simulink model "Rate_adaptivity"  (R2022a)
settings: Solver=FixedStepAuto  StartTime=0.0  StopTime=10.0  FixedStep=1e-3  RelTol=1e-3  EnableMultiTasking=on
undefined symbols (not defined in the file): D0, D1, magnitude, PTC16, PTC17
libraries: etargetslib x30, frdmk64flib x5, dspstat3 x1, simulink x1
settings Model: ExtModeTrigDuration=5  Creator=12791  LastModifiedBy=simll
settings OptimizationCC: EnhancedBackFolding=on  PassReuseOutputArgsAs=Individual arguments  ZeroExternalMemoryAtStartup=off  ZeroInternalMemoryAtStartup=off  MaxStackSize=64  OptimizeBlockOrder=speed  DifferentSizesBufferReuse=on  OptimizationCustomize=off  EfficientTunableParamExpr=on
settings DebuggingCC: ParameterTunabilityLossMsg=error
settings HardwareCC: ProdBitPerPointer=32  ProdBitPerSizeT=32  ProdBitPerPtrDiffT=32  ProdLargestAtomicInteger=Long  ProdLargestAtomicFloat=Double  ProdWordSize=32  ProdHWDeviceType=ARM Compatible->ARM Cortex
settings SFSimCC: MATLABDynamicMemAlloc=off
settings RTWCC: SystemTargetFile=ert.tlc  HardwareBoard=NXP FRDM-K64F  TLCOptions="-aInlineSetEventsForThisBaseRateFcn=TLC_FALSE -aSuppressMultiTaskScheduler=TLC_FALSE  -aRateBasedStepFcn=0"  TemplateMakefile=ert_default_tmf  Toolchain=GNU Tools for ARM Embedded Processors
settings CodeAppCC: ForceParamTrailComments=on  IgnoreCustomStorageClasses=off  OperatorAnnotations=on  SimulinkDataObjDesc=on  SFDataObjDesc=on  InsertBlockDesc=on
settings ERTTargetCC: ExtModeTransport=4  ExtModeMexFile=sendToCommService

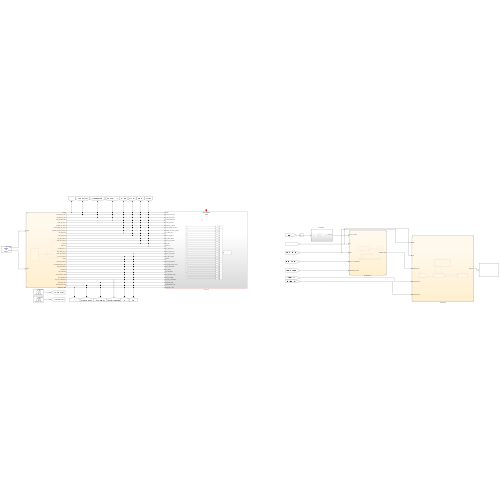
[thumbnail: Simulink's stored preview of the top-level diagram]
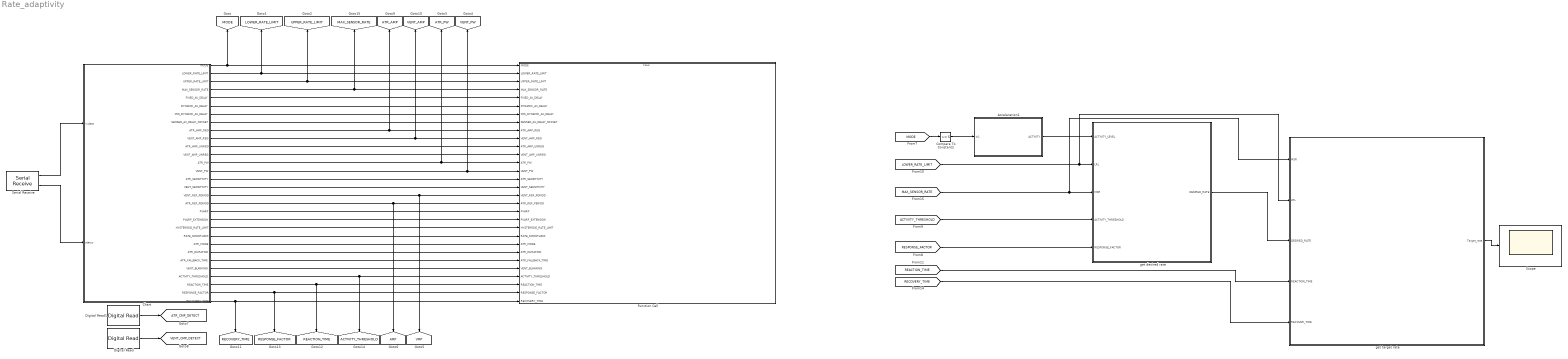
== system Rate_adaptivity ==
  Acceleration1 : Subsystem
  Chart : Stateflow chart  TreatAsAtomicUnit=on
  Compare To Constant2 : simulink/Logic and Bit Operations/Compare To Constant  relop=>=  const=5  OutDataTypeStr=boolean
  Digital Read : frdmk64flib/Digital Read  Whichpin=PTC17 (D1)  SampleTime=-1
  Digital Read1 : frdmk64flib/Digital Read  Whichpin=PTC16 (D0)  SampleTime=-1
  Function Call : Subsystem  TreatAsAtomicUnit=on
  Scope : Scope
  Serial Receive : frdmk64flib/Serial Receive  SCIModule=0  Baudrate=uint32(9600)  Parity=None  StopBits=1  HardwareFlowControl=None  ByteOrder=LittleEndian  DataType=uint8  DataLength=10  BlockingMode=off  OutputStatus=on  SampleTime=0.1
  get desired rate : Stateflow chart  TreatAsAtomicUnit=on
  get target rate : Stateflow chart  TreatAsAtomicUnit=on
      settings: PortSchema="{\"entries\":[{\"content\":{\"sides\":[{\"content\":{\"connectorIds\":[\"In3\",\"In2\",\"In1\",\"In4\",\"In5\"]},\"type\":\"ConnectorPlacement.EquallySpacedRectSide\",\"uuid\":\"b1115713-3752-47d5-be72-104b51cdb1c5\"},{\"content\":{\"connectorIds\":[\"Out1\"],\"side\":\"RIGHT\"},\"type\":\"ConnectorPlacement.EquallySpacedRectSide\",\"uuid\":\"0930a30a-8aa5-4912-ba1f-cc7f148656b0\"},{\"content\":{\"connectorIds\":[],\"side\":\"TOP\"},\"type\":\"ConnectorPlacement.EquallySpacedRectSide\",\"uuid\":\"94dfeeb6-c083-4dc2-b4f5-32fe99d16bb7\"}]},\"type\":\"ConnectorPlacement.EquallySpacedConnector\",\"uuid\":\"5d93a560-4d98-406a-ad12-5273aac4a25c\"}],\"packageUris\":[\"http://schema.mathworks.com/mf0/Connector/R2020b\"],\"version\":\"1.0\"}"
  tag scope: ACTIVITY_THRESHOLD=global, ARP=global, ATR_AMP=global, ATR_CMP_DETECT=global, ATR_PW=global, LOWER_RATE_LIMIT=global, MAX_SENSOR_RATE=global, MODE=global, REACTION_TIME=global, RECOVERY_TIME=global, RESPONSE_FACTOR=global, UPPER_RATE_LIMIT=global, VENT_AMP=global, VENT_CMP_DETECT=global, VENT_PW=global, VRP=global
  wires:
  Serial Receive/1 -> Chart/1(rxdata)
  Serial Receive/2 -> Chart/2(status)
  Chart/1(MODE) -> Function Call/1(MODE), [MODE]
  Chart/2(LOWER_RATE_LIMIT) -> Function Call/2(LOWER_RATE_LIMIT), [LOWER_RATE_LIMIT]
  Chart/3(UPPER_RATE_LIMIT) -> Function Call/3(UPPER_RATE_LIMIT), [UPPER_RATE_LIMIT]
  Chart/4(MAX_SENSOR_RATE) -> Function Call/4(MAX_SENSOR_RATE), [MAX_SENSOR_RATE]
  Chart/5(FIXED_AV_DELAY) -> Function Call/5(FIXED_AV_DELAY)
  Chart/6(DYNAMIC_AV_DELAY) -> Function Call/6(DYNAMIC_AV_DELAY)
  Chart/7(MIN_DYNAMIC_AV_DELAY) -> Function Call/7(MIN_DYNAMIC_AV_DELAY)
  Chart/8(SENSED_AV_DELAY_OFFSET) -> Function Call/8(SENSED_AV_DELAY_OFFSET)
  Chart/11(ATR_AMP_UNREG) -> Function Call/11(ATR_AMP_UNREG)
  Chart/12(VENT_AMP_UNREG) -> Function Call/12(VENT_AMP_UNREG)
  Chart/13(ATR_PW) -> Function Call/13(ATR_PW), [ATR_PW]
  Chart/14(VENT_PW) -> Function Call/14(VENT_PW), [VENT_PW]
  Chart/15(ATR_SENSITIVITY) -> Function Call/15(ATR_SENSITIVITY)
  Chart/16(VENT_SENSITIVITY) -> Function Call/16(VENT_SENSITIVITY)
  Chart/17(VENT_REF_PERIOD) -> Function Call/17(VENT_REF_PERIOD), [VRP]
  Chart/18(ATR_REF_PERIOD) -> Function Call/18(ATR_REF_PERIOD), [ARP]
  Chart/19(PVARP) -> Function Call/19(PVARP)
  Chart/20(PVARP_EXTENSION) -> Function Call/20(PVARP_EXTENSION)
  Chart/21(HYSTERESIS_RATE_LIMIT) -> Function Call/21(HYSTERESIS_RATE_LIMIT)
  Chart/22(RATE_SMOOTHING) -> Function Call/22(RATE_SMOOTHING)
  Chart/23(ATR_MODE) -> Function Call/23(ATR_MODE)
  Chart/24(ATR_DURATION) -> Function Call/24(ATR_DURATION)
  Chart/25(ATR_FALLBACK_TIME) -> Function Call/25(ATR_FALLBACK_TIME)
  Chart/26(VENT_BLANKING) -> Function Call/26(VENT_BLANKING)
  Chart/27(ACTIVITY_THRESHOLD) -> [ACTIVITY_THRESHOLD], Function Call/27(ACTIVITY_THRESHOLD)
  Chart/29(RESPONSE_FACTOR) -> Function Call/29(RESPONSE_FACTOR), [RESPONSE_FACTOR]
  Chart/30(RECOVERY_TIME) -> Function Call/30(RECOVERY_TIME), [RECOVERY_TIME]
  Digital Read1/1 -> [ATR_CMP_DETECT]
  Digital Read/1 -> [VENT_CMP_DETECT]
  Chart/10(VENT_AMP_REG) -> Function Call/10(VENT_AMP_REG), [VENT_AMP]
  Chart/9(ATR_AMP_REG) -> Function Call/9(ATR_AMP_REG), [ATR_AMP]
  Chart/28(REACTION_TIME) -> Function Call/28(REACTION_TIME), [REACTION_TIME]
  [MODE] -> Compare To Constant2/1
  Compare To Constant2/1 -> Acceleration1/1(In1)
  Acceleration1/1(ACTIVITY) -> get desired rate/1(ACTIVITY_LEVEL)
  [LOWER_RATE_LIMIT] -> get desired rate/2(LRL), get target rate/2(LRL)
  [MAX_SENSOR_RATE] -> get desired rate/3(MSR), get target rate/3(MSR)
  [ACTIVITY_THRESHOLD] -> get desired rate/4(ACTIVITY_THRESHOLD)
  [RESPONSE_FACTOR] -> get desired rate/5(RESPONSE_FACTOR)
  get desired rate/1(DESIRED_RATE) -> get target rate/1(DESIRED_RATE)
  [REACTION_TIME] -> get target rate/4(REACTION_TIME)
  [RECOVERY_TIME] -> get target rate/5(RECOVER_TIME)
  get target rate/1(Target_rate) -> Scope/1

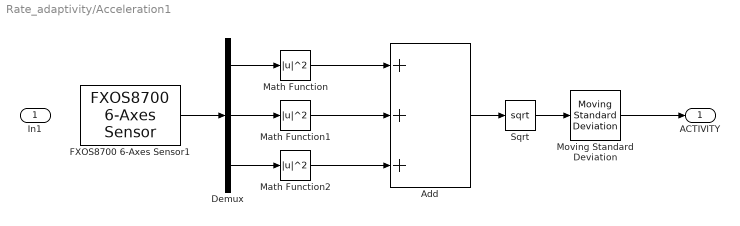
== system Rate_adaptivity/Acceleration1 ==
  In1 : Inport
  Add : Sum  Inputs=+++
  Demux : Demux  Outputs=3
  FXOS8700 6-Axes Sensor1 : frdmk64flib/FXOS8700 6-Axes Sensor  Activesensor=Accelerometer only  ODR=800Hz  HybridODR=400Hz  Accelfullrange=-4g to +4g  SampleTime=-1
  Math Function : Math  Operator=magnitude^2  SignedPower=on  OutDataTypeStr=double
  Math Function1 : Math  Operator=magnitude^2  SignedPower=on  OutDataTypeStr=double
  Math Function2 : Math  Operator=magnitude^2  SignedPower=on  OutDataTypeStr=double
  Moving Standard Deviation : dspstat3/Moving Standard Deviation  Method=Sliding window  ForgettingFactorPort=off  SpecifyWindowLength=on  WindowLength=4  ForgettingFactor=0.9  SimulateUsing=Code generation
      settings: SourceProductBaseCode=DS
  Sqrt : Sqrt
  ACTIVITY : Outport  SourceOfInitialOutputValue=Input signal
  wires:
  Sqrt/1 -> Moving Standard Deviation/1
  Math Function2/1 -> Add/3
  Add/1 -> Sqrt/1
  Math Function1/1 -> Add/2
  Demux/1 -> Math Function/1
  Demux/2 -> Math Function1/1
  Math Function/1 -> Add/1
  FXOS8700 6-Axes Sensor1/1 -> Demux/1
  Demux/3 -> Math Function2/1
  Moving Standard Deviation/1 -> ACTIVITY/1

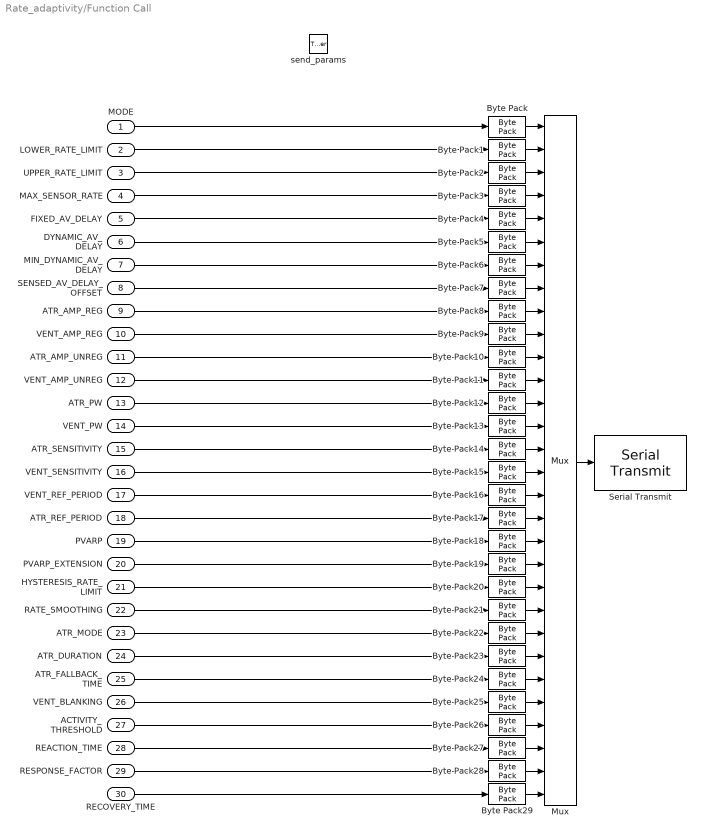
== system Rate_adaptivity/Function Call ==
  MODE : Inport
  LOWER_RATE_LIMIT : Inport  Port=2
  UPPER_RATE_LIMIT : Inport  Port=3
  MAX_SENSOR_RATE : Inport  Port=4
  FIXED_AV_DELAY : Inport  Port=5
  DYNAMIC_AV_DELAY : Inport  Port=6
  MIN_DYNAMIC_AV_DELAY : Inport  Port=7
  SENSED_AV_DELAY_OFFSET : Inport  Port=8
  ATR_AMP_REG : Inport  Port=9
  VENT_AMP_REG : Inport  Port=10
  ATR_AMP_UNREG : Inport  Port=11
  VENT_AMP_UNREG : Inport  Port=12
  ATR_PW : Inport  Port=13
  VENT_PW : Inport  Port=14
  ATR_SENSITIVITY : Inport  Port=15
  VENT_SENSITIVITY : Inport  Port=16
  VENT_REF_PERIOD : Inport  Port=17
  ATR_REF_PERIOD : Inport  Port=18
  PVARP : Inport  Port=19
  PVARP_EXTENSION : Inport  Port=20
  HYSTERESIS_RATE_LIMIT : Inport  Port=21
  RATE_SMOOTHING : Inport  Port=22
  ATR_MODE : Inport  Port=23
  ATR_DURATION : Inport  Port=24
  ATR_FALLBACK_TIME : Inport  Port=25
  VENT_BLANKING : Inport  Port=26
  ACTIVITY_THRESHOLD : Inport  Port=27
  REACTION_TIME : Inport  Port=28
  RESPONSE_FACTOR : Inport  Port=29
  RECOVERY_TIME : Inport  Port=30
  send_params : TriggerPort  TriggerType=function-call  IsSimulinkFunction=on  FunctionName=send_params  VariantControl=Variant
  Byte Pack{,1..4,6..7,16..21,23..25,27..29} (19 alike) : etargetslib/Byte Pack  datatypes={'uint16'}  byteAlign=1
  Byte Pack{8..15,26} (9 alike) : etargetslib/Byte Pack  datatypes={'double'}  byteAlign=1
  Byte Pack22 : etargetslib/Byte Pack  datatypes={'boolean'}  byteAlign=1
  Byte Pack5 : etargetslib/Byte Pack  datatypes={'boolean'}  byteAlign=1
  Mux : Mux  Inputs=30
  Serial Transmit : frdmk64flib/Serial Transmit  SCIModule=0  Baudrate=uint32(9600)  Parity=None  StopBits=1  HardwareFlowControl=None  ByteOrder=LittleEndian  BlockingMode=on  OutputStatus=off
  wires:
  PVARP/1 -> Byte Pack18/1
  ATR_SENSITIVITY/1 -> Byte Pack14/1
  PVARP_EXTENSION/1 -> Byte Pack19/1
  MAX_SENSOR_RATE/1 -> Byte Pack3/1
  Byte Pack1/1 -> Mux/2
  Byte Pack7/1 -> Mux/8
  Byte Pack21/1 -> Mux/22
  ATR_AMP_UNREG/1 -> Byte Pack10/1
  Byte Pack/1 -> Mux/1
  Byte Pack20/1 -> Mux/21
  Byte Pack22/1 -> Mux/23
  Byte Pack3/1 -> Mux/4
  Byte Pack18/1 -> Mux/19
  VENT_REF_PERIOD/1 -> Byte Pack16/1
  Byte Pack17/1 -> Mux/18
  Mux/1 -> Serial Transmit/1
  Byte Pack26/1 -> Mux/27
  Byte Pack12/1 -> Mux/13
  LOWER_RATE_LIMIT/1 -> Byte Pack1/1
  RECOVERY_TIME/1 -> Byte Pack29/1
  Byte Pack9/1 -> Mux/10
  Byte Pack19/1 -> Mux/20
  Byte Pack13/1 -> Mux/14
  RESPONSE_FACTOR/1 -> Byte Pack28/1
  ATR_DURATION/1 -> Byte Pack23/1
  RATE_SMOOTHING/1 -> Byte Pack21/1
  Byte Pack8/1 -> Mux/9
  REACTION_TIME/1 -> Byte Pack27/1
  Byte Pack29/1 -> Mux/30
  Byte Pack16/1 -> Mux/17
  Byte Pack25/1 -> Mux/26
  ATR_MODE/1 -> Byte Pack22/1
  VENT_SENSITIVITY/1 -> Byte Pack15/1
  Byte Pack11/1 -> Mux/12
  VENT_PW/1 -> Byte Pack13/1
  MODE/1 -> Byte Pack/1
  VENT_AMP_REG/1 -> Byte Pack9/1
  Byte Pack24/1 -> Mux/25
  Byte Pack15/1 -> Mux/16
  Byte Pack2/1 -> Mux/3
  MIN_DYNAMIC_AV_DELAY/1 -> Byte Pack6/1
  VENT_BLANKING/1 -> Byte Pack25/1
  Byte Pack28/1 -> Mux/29
  ATR_PW/1 -> Byte Pack12/1
  FIXED_AV_DELAY/1 -> Byte Pack4/1
  VENT_AMP_UNREG/1 -> Byte Pack11/1
  Byte Pack4/1 -> Mux/5
  UPPER_RATE_LIMIT/1 -> Byte Pack2/1
  Byte Pack27/1 -> Mux/28
  SENSED_AV_DELAY_OFFSET/1 -> Byte Pack7/1
  Byte Pack6/1 -> Mux/7
  ATR_AMP_REG/1 -> Byte Pack8/1
  Byte Pack14/1 -> Mux/15
  Byte Pack10/1 -> Mux/11
  DYNAMIC_AV_DELAY/1 -> Byte Pack5/1
  Byte Pack5/1 -> Mux/6
  ATR_REF_PERIOD/1 -> Byte Pack17/1
  ACTIVITY_THRESHOLD/1 -> Byte Pack26/1
  Byte Pack23/1 -> Mux/24
  HYSTERESIS_RATE_LIMIT/1 -> Byte Pack20/1
  ATR_FALLBACK_TIME/1 -> Byte Pack24/1

== stateflow chart Rate_adaptivity/get desired rate ==
  state check
    %check if the actvity level below the threshold
  state Desires_output_1
    entry:
    DESIRED_RATE=LRL;
  state Desires_output_3
    entry:
    DESIRED_RATE = Local_rate;
  state Desires_output_2
    entry:
    DESIRED_RATE = MSR;
  state Increase_Linear
    entry:
    Local_rate = LRL + RESPONSE_FACTOR*(ACTIVITY_LEVEL-ACTIVITY_THRESHOLD);
  (default) -> check
  check -> Desires_output_1 [order 1] : [ACTIVITY_LEVEL<=ACTIVITY_THRESHOLD]
  Desires_output_1 -> check : after(100,msec)
  check -> Increase_Linear [order 2] : [ACTIVITY_LEVEL>ACTIVITY_THRESHOLD]
  Desires_output_3 -> check : after(100,msec)
  Desires_output_2 -> check : after(100,msec)
  Increase_Linear -> Desires_output_2 [order 1] : [Local_rate >=MSR]
  Increase_Linear -> Desires_output_3 [order 2] : [Local_rate<MSR]
  data: ACTIVITY_LEVEL input; LRL input; MSR input; ACTIVITY_THRESHOLD input; RESPONSE_FACTOR input; DESIRED_RATE output; Local_rate local

== stateflow chart Rate_adaptivity/get target rate ==
  state increase_state
    entry:
    %use linear:
    if(Target_rate<MSR && Target_rate<DESIRED_RATE)
    Target_rate=Target_rate+step_up;
    elseif(Target_rate == DESIRED_RATE)
    Target_rate = DESIRED_RATE;
    elseif(Target_rate>MSR)
    Target_rate = MSR
    end
  state step_state
    entry:
    step_up = (MSR-LRL)/REACTION_TIME;
    step_down = (MSR-LRL)/RECOVER_TIME;
  state decrease_state
    entry:
    if(Target_rate<MSR)
    Target_rate = Target_rate - step_down;
    elseif(Target_rate <= LRL)
    Target_rate = LRL;
    end
  state start_state
    %set target rate to at least LRL
    Target_rate = LRL;
  step_state -> increase_state [order 2] : after(100,msec)[Target_rate<=DESIRED_RATE]
  increase_state -> step_state : after(100,msec)
  (default) -> start_state
  step_state -> decrease_state [order 1] : after(100,msec)[Target_rate>DESIRED_RATE]
  decrease_state -> step_state : after(100,msec)
  start_state -> step_state : [Target_rate>=LRL]
  data: DESIRED_RATE input; Target_rate output; LRL input; MSR input; REACTION_TIME input; RECOVER_TIME input; step_down local; step_up local

== stateflow chart Rate_adaptivity/Chart ==
  settings: executeAtInitialization=1
  state SET_PARAM
    entry:
    MODE = 6;
    LOWER_RATE_LIMIT = typecast(rxdata(3:4), 'uint16'); % ppm
    UPPER_RATE_LIMIT = typecast(rxdata(5:6), 'uint16'); % ppm
    MAX_SENSOR_RATE = typecast(rxdata(7:8), 'uint16'); % ppm
    FIXED_AV_DELAY = typecast(rxdata(9:10), 'uint16'); % ms
    DYNAMIC_AV_DELAY = rxdata(11); % boolean
    MIN_DYNAMIC_AV_DELAY =  typecast(rxdata(12:13), 'uint16'); % ms
    SENSED_AV_DELAY_OFFSET = typecast(rxdata(14:15), 'uint16'); % ms
    ATR_AMP_REG =  typecast(rxdata(9:16), 'double'); % V
    VENT_AMP_REG = typecast(rxdata(9:16), 'double'); % V
    ATR_AMP_UNREG = typecast(rxdata(9:16), 'double'); % V
    VENT_AMP_UNREG = typecast(rxdata(9:16), 'double'); % V
    ATR_PW = typecast(rxdata(9:16), 'double'); % ms
    VENT_PW = typecast(rxdata(9:16), 'double'); % ms
    ATR_SENSITIVITY = typecast(rxdata(9:16), 'double'); % mV
    VENT_SENSITIVITY = typecast(rxdata(9:16), 'double'); % mV
    VENT_REF_PERIOD = typecast(rxdata(14:15), 'uint16'); % ms
    ATR_REF_PERIOD = typecast(rxdata(14:15), 'uint16'); % ms
    PVARP = typecast(rxdata(14:15), 'uint16'); % ms
    PVARP_EXTENSION = typecast(rxdata(14:15), 'uint16'); % ms
    HYSTERESIS_RATE_LIMIT = typecast(rxdata(14:15), 'uint16'); % ms
    RATE_SMOOTHING = typecast(rxdata(14:15), 'uint16'); % percentage
    ATR_MODE = rxdata(14); % boolean
    ATR_DURATION = typecast(rxdata(14:15), 'uint16'); % cc
    ATR_FALLBACK_TIME = typecast(rxdata(14:15), 'uint16'); % min
    VENT_BLANKING = typecast(rxdata(14:15), 'uint16'); % ms
    ACTIVITY_THRESHOLD = typecast(rxdata(14:15), 'uint16');
    REACTION_TIME = typecast(rxdata(14:15), 'uint16'); % s
    RESPONSE_FACTOR = typecast(rxdata(14:15), 'uint16');
    RECOVERY_TIME = typecast(rxdata(14:15), 'uint16'); % min
  state INITIAL
    % Set the initial values of parameters
    entry:
    MODE = 6;
    LOWER_RATE_LIMIT = 60; % ppm
    UPPER_RATE_LIMIT = 120; % ppm
    MAX_SENSOR_RATE = 120; % ppm
    FIXED_AV_DELAY = 150; % ms
    DYNAMIC_AV_DELAY = false; % boolean
    MIN_DYNAMIC_AV_DELAY = 50; % ms
    SENSED_AV_DELAY_OFFSET = 0; % ms
    ATR_AMP_REG = 3.5; % V
    VENT_AMP_REG = 3.5; % V
    ATR_AMP_UNREG = 3.75; % V
    VENT_AMP_UNREG = 3.75; % V
    ATR_PW = 0.4; % ms
    VENT_PW = 0.4; % ms
    ATR_SENSITIVITY = 0.75; % mV
    VENT_SENSITIVITY = 2.5; % mV
    VENT_REF_PERIOD = 320; % ms
    ATR_REF_PERIOD = 250; % ms
    PVARP = 250; % ms
    PVARP_EXTENSION = 0; % ms
    HYSTERESIS_RATE_LIMIT = 0; % ms
    RATE_SMOOTHING = 0; % percentage
    ATR_MODE = false; % boolean
    ATR_DURATION = 20; % cc
    ATR_FALLBACK_TIME = 1; % min
    VENT_BLANKING = 40; % ms
    ACTIVITY_THRESHOLD = 0;
    REACTION_TIME = 30; % s
    RESPONSE_FACTOR = 8;
    RECOVERY_TIME = 5; % min
  state STANDBY
    %Waiting for COM
  state ECHO_PARAM
    entry:
    send_params();
  SET_PARAM -> STANDBY
  (default) -> INITIAL
  (junction 16) -> SET_PARAM [order 1] : [rxdata(2) == hex2dec('55')]
  (junction 13) -> STANDBY [order 2]
  INITIAL -> STANDBY
  STANDBY -> (junction 13) : [status == 0]
  (junction 13) -> (junction 16) [order 1] : [rxdata(1) == hex2dec('16')]
  (junction 16) -> ECHO_PARAM [order 2] : [rxdata(2) == hex2dec('22')]
  ECHO_PARAM -> STANDBY
  data: rxdata input; status input; MODE output; LOWER_RATE_LIMIT output; UPPER_RATE_LIMIT output; MAX_SENSOR_RATE output; FIXED_AV_DELAY output; DYNAMIC_AV_DELAY output; MIN_DYNAMIC_AV_DELAY output; SENSED_AV_DELAY_OFFSET output; ATR_AMP_REG output; VENT_AMP_REG output; ATR_AMP_UNREG output; VENT_AMP_UNREG output; ATR_PW output; VENT_PW output; ATR_SENSITIVITY output; VENT_SENSITIVITY output; VENT_REF_PERIOD output; ATR_REF_PERIOD output; PVARP output; PVARP_EXTENSION output; HYSTERESIS_RATE_LIMIT output; RATE_SMOOTHING output; ATR_MODE output; ATR_DURATION output; ATR_FALLBACK_TIME output; VENT_BLANKING output; ACTIVITY_THRESHOLD output; REACTION_TIME output; RESPONSE_FACTOR output; RECOVERY_TIME output
